simulink model "EST"  (R2023b)
settings: Solver=FixedStepAuto  StartTime=0.0  StopTime=stopt  FixedStep=deltat  MaxStep=0.05  RelTol=1e-3
InitFcn:
  | clear all;
  | close all;
  | clc;
  | 
  | % add the data and script directories
  | addpath('data','scripts');
  | 
  | % load the constants (units)
  | constants;
  | 
  | % load the simulation parameters
  | preprocessing;
StopFcn:
  | postprocessing;
values from neighbouring files (symbols this model uses):
  aElectricityDemandTransport = 0.01    [preprocessing.m]
  aExtraction = efficiency    [preprocessing.m]
  aHeatingDemandTransport = 0.01    [preprocessing.m]
  COP65 = 3    [preprocessing.m]
  COP80 = 2.48    [preprocessing.m]
  diameter = 1.2    [preprocessing.m]
  EStorageInitial = 10^5    (= 100000)    [preprocessing.m]
  EStorageMax = Tmax*HeatCapacity    (= 469413657.839)    [preprocessing.m]
  EStorageMin = Tmin*HeatCapacity    (= 352060243.38)    [preprocessing.m]
  HeatCapacity = WaterMass * SpecificHeat    (= 5867670.72299)    [preprocessing.m]
  HeatTransferCoefficient = 0.48    [preprocessing.m]
  InsulationThickness = 0.05    [preprocessing.m]
  SupplyVoltage = 230    [preprocessing.m]
  SupplyWireRestance = (WireLenght * ElectricalConductivity) / SupplyWireArea    (= 0.00530083402298)    [preprocessing.m]
  Tambient = 20    [preprocessing.m]
settings Model: Creator=joche  LastModifiedBy=20244239
settings DataIOCC: SaveFormat=Array  SaveOutput=off  ReturnWorkspaceOutputs=off
settings OptimizationCC: ReuseModelBlockBuffer=off
settings ModelReferenceCC: EnableRefExpFcnMdlSchedulingChecks=on

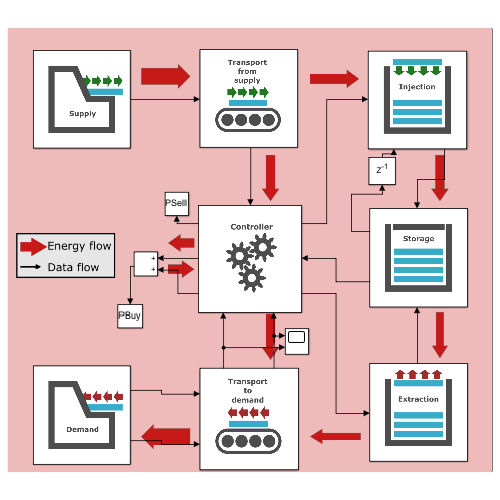
[thumbnail: Simulink's stored preview of the top-level diagram]
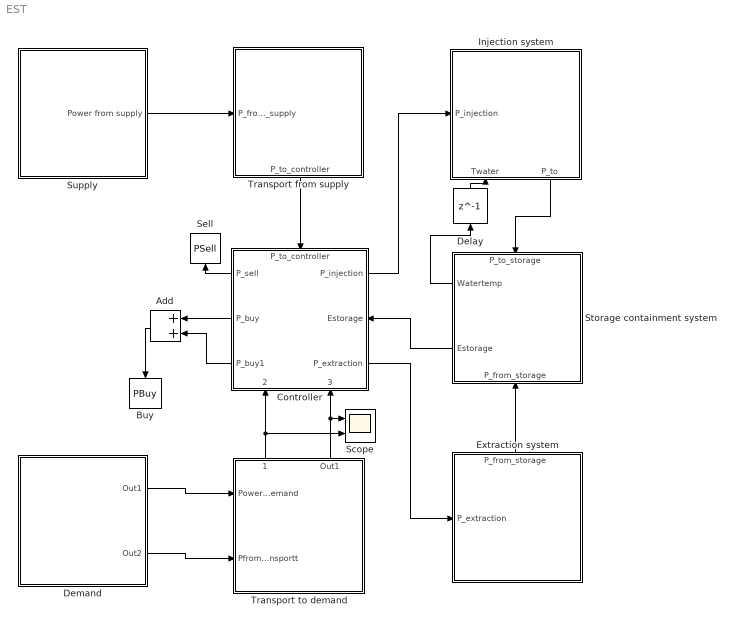
== system EST ==
  Add : Sum
  Buy : ToWorkspace  VariableName=PBuy  SampleTime=-1
  Controller : Subsystem
      settings: PortSchema="{\"entries\":[{\"content\":{\"sides\":[{\"content\":{\"connectorIds\":[\"Out3\",\"Out4\",\"Out5\"]},\"type\":\"ConnectorPlacement.EquallySpacedRectSide\",\"uuid\":\"4daf33ce-c96a-4783-b5c4-228eed953e01\"},{\"content\":{\"connectorIds\":[\"Out1\",\"In4\",\"Out2\"],\"side\":\"RIGHT\"},\"type\":\"ConnectorPlacement.EquallySpacedRectSide\",\"uuid\":\"e9942e50-8467-4af8-b79b-80636cbc76e5\"},{\"content\":{\"connectorIds\":[\"In1\"],\"side\":\"TOP\"},\"type\":\"ConnectorPlacement.EquallySpacedRectSide\",\"uuid\":\"f315e931-d69b-4751-b712-f89c6c81baeb\"},{\"content\":{\"connectorIds\":[\"In2\",\"In3\"],\"side\":\"BOTTOM\"},\"type\":\"ConnectorPlacement.EquallySpacedRectSide\",\"uuid\":\"44715ee6-5cd5-4669-bcb9-5ed7c869bdb3\"}]},\"type\":\"ConnectorPlacement.EquallySpacedConnector\",\"uuid\":\"fff48899-944b-4064-b7d7-ecc12144fb48\"}],\"packageUris\":[\"http://schema.mathworks.com/mf0/Connector/R2020b\"],\"version\":\"1.0\"}"
      mask Display: image('$imagefile'); % Use "Edit Image" on toolstrip to change.
  Delay : Delay  DelayLength=1  InitialCondition=0
  Demand : Subsystem
      mask Display: image('$imagefile'); % Use "Edit Image" on toolstrip to change.
  Extraction system : Subsystem
      settings: PortSchema="{\"entries\":[{\"content\":{\"sides\":[{\"content\":{\"connectorIds\":[]},\"type\":\"ConnectorPlacement.EquallySpacedRectSide\",\"uuid\":\"05c5933d-55fc-4e06-853f-fc26d42905f9\"},{\"content\":{\"connectorIds\":[\"In1\"],\"side\":\"RIGHT\"},\"type\":\"ConnectorPlacement.EquallySpacedRectSide\",\"uuid\":\"327426c5-31d5-498b-a2bd-83e49353408c\"},{\"content\":{\"connectorIds\":[],\"side\":\"TOP\"},\"type\":\"ConnectorPlacement.EquallySpacedRectSide\",\"uuid\":\"55306cf3-a3de-4385-a5ae-b8600ecdd5a2\"},{\"content\":{\"connectorIds\":[\"Out1\"],\"side\":\"BOTTOM\"},\"type\":\"ConnectorPlacement.EquallySpacedRectSide\",\"uuid\":\"08fcc9c3-40d3-4ac6-b914-dfeef6039ffb\"}]},\"type\":\"ConnectorPlacement.EquallySpacedConnector\",\"uuid\":\"cb35d5ba-e8c6-462c-b7b2-fe8356d4b0a1\"}],\"packageUris\":[\"http://schema.mathworks.com/mf0/Connector/R2020b\"],\"version\":\"1.0\"}"
      mask Display: image('$imagefile'); % Use "Edit Image" on toolstrip to change.
  Injection system : Subsystem
      settings: PortSchema="{\"entries\":[{\"content\":{\"sides\":[{\"content\":{},\"type\":\"ConnectorPlacement.EquallySpacedRectSide\",\"uuid\":\"05c5933d-55fc-4e06-853f-fc26d42905f9\"},{\"content\":{\"connectorIds\":[\"In2\"],\"side\":\"RIGHT\"},\"type\":\"ConnectorPlacement.EquallySpacedRectSide\",\"uuid\":\"327426c5-31d5-498b-a2bd-83e49353408c\"},{\"content\":{\"connectorIds\":[\"Out1\",\"In1\"],\"side\":\"TOP\"},\"type\":\"ConnectorPlacement.EquallySpacedRectSide\",\"uuid\":\"55306cf3-a3de-4385-a5ae-b8600ecdd5a2\"},{\"content\":{\"side\":\"BOTTOM\"},\"type\":\"ConnectorPlacement.EquallySpacedRectSide\",\"uuid\":\"08fcc9c3-40d3-4ac6-b914-dfeef6039ffb\"}]},\"type\":\"ConnectorPlacement.EquallySpacedConnector\",\"uuid\":\"cb35d5ba-e8c6-462c-b7b2-fe8356d4b0a1\"}],\"packageUris\":[\"http://schema.mathworks.com/mf0/Connector/R2020b\"],\"version\":\"1.0\"}"
      mask Display: image('$imagefile'); % Use "Edit Image" on toolstrip to change.
  Scope : Scope  NumInputPorts=2
  Sell : ToWorkspace  VariableName=PSell  SampleTime=-1
  Storage containment system : Subsystem
      settings: PortSchema="{\"entries\":[{\"content\":{\"sides\":[{\"content\":{\"connectorIds\":[\"Out1\",\"Out2\"]},\"type\":\"ConnectorPlacement.EquallySpacedRectSide\",\"uuid\":\"0ba48424-33b9-4934-970f-64fe5d8b070e\"},{\"content\":{\"side\":\"RIGHT\"},\"type\":\"ConnectorPlacement.EquallySpacedRectSide\",\"uuid\":\"9cde340f-8f39-4499-9a12-5e1623737660\"},{\"content\":{\"connectorIds\":[\"In1\"],\"side\":\"TOP\"},\"type\":\"ConnectorPlacement.EquallySpacedRectSide\",\"uuid\":\"2af8db04-7fd0-4902-8637-8dc00edb4598\"},{\"content\":{\"connectorIds\":[\"In2\"],\"side\":\"BOTTOM\"},\"type\":\"ConnectorPlacement.EquallySpacedRectSide\",\"uuid\":\"e21ea806-d777-41a3-a53f-556fae66854b\"}]},\"type\":\"ConnectorPlacement.EquallySpacedConnector\",\"uuid\":\"4e2ddb36-4db3-4ab4-858b-ebb8ccefeb1f\"}],\"packageUris\":[\"http://schema.mathworks.com/mf0/Connector/R2020b\"],\"version\":\"1.0\"}"
      mask Display: image('$imagefile'); % Use "Edit Image" on toolstrip to change.
  Supply : Subsystem
      mask Display: image('$imagefile'); % Use "Edit Image" on toolstrip to change.
  Transport from supply : Subsystem
      settings: PortSchema="{\"entries\":[{\"content\":{\"sides\":[{\"content\":{\"connectorIds\":[\"In1\"]},\"type\":\"ConnectorPlacement.EquallySpacedRectSide\",\"uuid\":\"31329006-3d36-4d93-9c44-7503a515d397\"},{\"content\":{\"connectorIds\":[],\"side\":\"RIGHT\"},\"type\":\"ConnectorPlacement.EquallySpacedRectSide\",\"uuid\":\"aba139c7-f9b6-4881-a56b-a4cbbedacd88\"},{\"content\":{\"connectorIds\":[],\"side\":\"TOP\"},\"type\":\"ConnectorPlacement.EquallySpacedRectSide\",\"uuid\":\"e683eb73-7a35-4160-9c39-da83856a6278\"},{\"content\":{\"connectorIds\":[\"Out1\"],\"side\":\"BOTTOM\"},\"type\":\"ConnectorPlacement.EquallySpacedRectSide\",\"uuid\":\"1170dd18-447c-437f-9043-6812c2877331\"}]},\"type\":\"ConnectorPlacement.EquallySpacedConnector\",\"uuid\":\"804af608-1d70-444f-af69-e05f19bf98f3\"}],\"packageUris\":[\"http://schema.mathworks.com/mf0/Connector/R2020b\"],\"version\":\"1.0\"}"
      mask Display: image('$imagefile'); % Use "Edit Image" on toolstrip to change.
  Transport to demand : Subsystem
      settings: PortSchema="{\"entries\":[{\"content\":{\"sides\":[{\"content\":{\"connectorIds\":[\"In1\",\"In2\"]},\"type\":\"ConnectorPlacement.EquallySpacedRectSide\",\"uuid\":\"03dcb471-e366-4ed9-a75b-6b53ae3db544\"},{\"content\":{\"side\":\"RIGHT\"},\"type\":\"ConnectorPlacement.EquallySpacedRectSide\",\"uuid\":\"6dd80e9d-b764-41ba-981e-efa62bb14601\"},{\"content\":{\"connectorIds\":[\"Out1\",\"Out2\"],\"side\":\"TOP\"},\"type\":\"ConnectorPlacement.EquallySpacedRectSide\",\"uuid\":\"5418711a-b225-492f-884c-10526dc9bc30\"}]},\"type\":\"ConnectorPlacement.EquallySpacedConnector\",\"uuid\":\"979ac05e-7956-4b8d-8463-5f461851369c\"}],\"packageUris\":[\"http://schema.mathworks.com/mf0/Connector/R2020b\"],\"version\":\"1.0\"}"
      mask Display: image('$imagefile'); % Use "Edit Image" on toolstrip to change.
  wires:
  Supply/1(Power from supply) -> Transport from supply/1(P_from_supply)
  Transport from supply/1(P_to_controller) -> Controller/1(P_to_controller)
  Transport to demand/1(P_from_controler) -> Scope/2, Controller/2(P_from_controller)
  Demand/1(Out1) -> Transport to demand/1(Power to demand)
  Controller/3(P_sell) -> Sell/1
  Controller/2(P_extraction) -> Extraction system/1(P_extraction)
  Injection system/1(P_to) -> Storage containment system/1(P_to_storage)
  Extraction system/1(P_from_storage) -> Storage containment system/2(P_from_storage)
  Controller/1(P_injection) -> Injection system/2(P_injection)
  Controller/4(P_buy) -> Add/1
  Demand/2(Out2) -> Transport to demand/2(PfromElectricityDemandTransportt)
  Transport to demand/2(Out1) -> Controller/3(PElectricityFromController), Scope/1
  Controller/5(P_buy1) -> Add/2
  Add/1 -> Buy/1
  Storage containment system/2(Estorage) -> Controller/4(Estorage)
  Storage containment system/1(Watertemp) -> Delay/1
  Delay/1 -> Injection system/1(Twater)

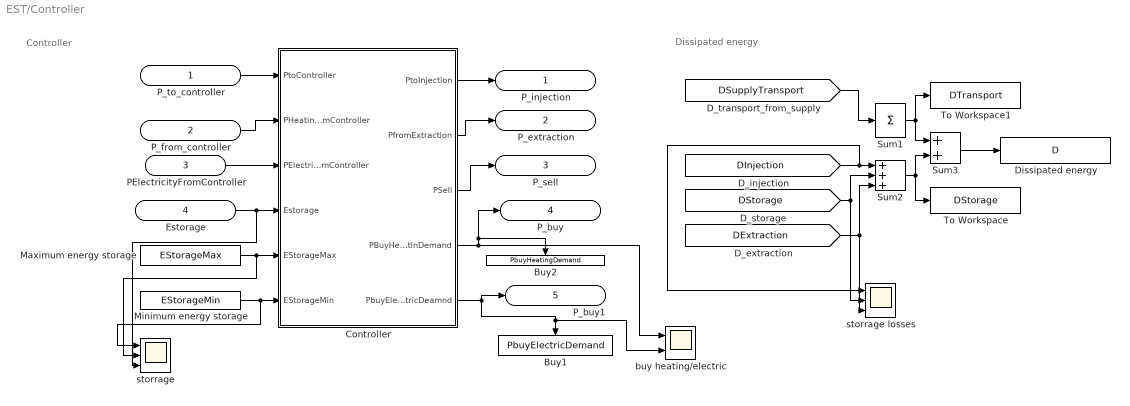
== system EST/Controller ==
  note: Dissipated energy
  note: Controller
  P_to_controller : Inport
  P_from_controller : Inport  Port=2
  PElectricityFromController : Inport  Port=3
  Estorage : Inport  Port=4
  Buy1 : ToWorkspace  VariableName=PbuyElectricDemand  SampleTime=-1
  Buy2 : ToWorkspace  VariableName=PbuyHeatingDemand  SampleTime=-1
  Controller : MATLAB Function  TreatAsAtomicUnit=on
  Dissipated energy : ToWorkspace  VariableName=D  SampleTime=-1
  Maximum energy storage : Constant  Value=EStorageMax
  Minimum energy storage : Constant  Value=EStorageMin
  Sum1 : Sum  Inputs=+
  Sum2 : Sum  Inputs=+++
  Sum3 : Sum
  To Workspace : ToWorkspace  VariableName=DStorage  SampleTime=-1
  To Workspace1 : ToWorkspace  VariableName=DTransport  SampleTime=-1
  buy heating/electric : Scope  NumInputPorts=2
  storrage : Scope  NumInputPorts=3
  storrage losses : Scope  NumInputPorts=3
  P_injection : Outport
  P_extraction : Outport  Port=2
  P_sell : Outport  Port=3
  P_buy : Outport  Port=4
  P_buy1 : Outport  Port=5
  wires:
  P_from_controller/1 -> Controller/2(PHeatingfromController)
  Controller/2(PfromExtraction) -> P_extraction/1
  Controller/3(PSell) -> P_sell/1
  Controller/4(PBuyHeatinDemand) -> buy heating/electric/1, P_buy/1, Buy2/1
  Minimum energy storage/1 -> storrage/1, Controller/6(EStorageMin)
  Maximum energy storage/1 -> storrage/2, Controller/5(EStorageMax)
  P_to_controller/1 -> Controller/1(PtoController)
  Controller/1(PtoInjection) -> P_injection/1
  Estorage/1 -> storrage/3, Controller/4(Estorage)
  [DSupplyTransport] -> Sum1/1
  [DInjection] -> storrage losses/1, Sum2/1
  [DStorage] -> Sum2/2, storrage losses/2
  [DExtraction] -> Sum2/3, storrage losses/3
  Sum2/1 -> To Workspace/1, Sum3/2
  Sum1/1 -> To Workspace1/1, Sum3/1
  Sum3/1 -> Dissipated energy/1
  PElectricityFromController/1 -> Controller/3(PElectricityFromController)
  Controller/5(PbuyElectricDeamnd) -> buy heating/electric/2, Buy1/1, P_buy1/1

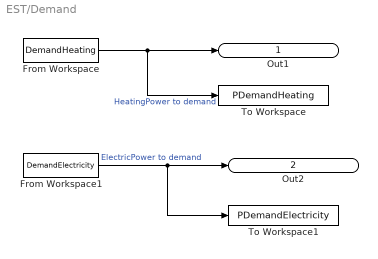
== system EST/Demand ==
  From Workspace : FromWorkspace  VariableName=DemandHeating  OutputAfterFinalValue=Setting to zero
  From Workspace1 : FromWorkspace  VariableName=DemandElectricity  OutputAfterFinalValue=Setting to zero
  To Workspace : ToWorkspace  VariableName=PDemandHeating  SampleTime=-1
  To Workspace1 : ToWorkspace  VariableName=PDemandElectricity  SampleTime=-1
  Out1 : Outport
  Out2 : Outport  Port=2
  wires:
  From Workspace/1 -> To Workspace/1, Out1/1  "HeatingPower to demand"
  From Workspace1/1 -> To Workspace1/1, Out2/1  "ElectricPower to demand"

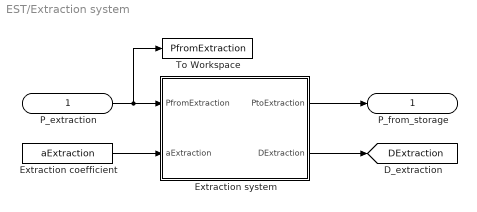
== system EST/Extraction system ==
  P_extraction : Inport
  Extraction coefficient : Constant  Value=aExtraction
  Extraction system : MATLAB Function  TreatAsAtomicUnit=on
  To Workspace : ToWorkspace  VariableName=PfromExtraction  SampleTime=-1
  P_from_storage : Outport
  tag scope: DExtraction=global
  wires:
  P_extraction/1 -> To Workspace/1, Extraction system/1(PfromExtraction)
  Extraction system/1(PtoExtraction) -> P_from_storage/1
  Extraction coefficient/1 -> Extraction system/2(aExtraction)
  Extraction system/2(DExtraction) -> [DExtraction]

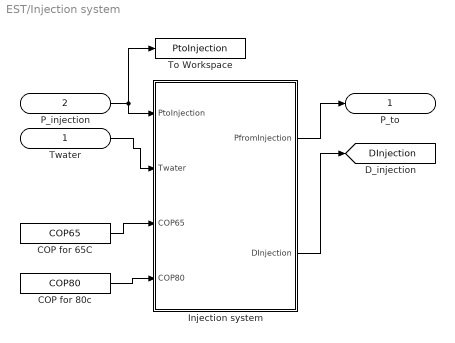
== system EST/Injection system ==
  Twater : Inport
  P_injection : Inport  Port=2
  COP for 65C : Constant  Value=COP65
  COP for 80c : Constant  Value=COP80
  Injection system : MATLAB Function  TreatAsAtomicUnit=on
  To Workspace : ToWorkspace  VariableName=PtoInjection  SampleTime=-1
  P_to : Outport
  tag scope: DInjection=global
  wires:
  P_injection/1 -> To Workspace/1, Injection system/1(PtoInjection)
  Injection system/1(PfromInjection) -> P_to/1
  Injection system/2(DInjection) -> [DInjection]
  COP for 65C/1 -> Injection system/3(COP65)
  COP for 80c/1 -> Injection system/4(COP80)
  Twater/1 -> Injection system/2(Twater)

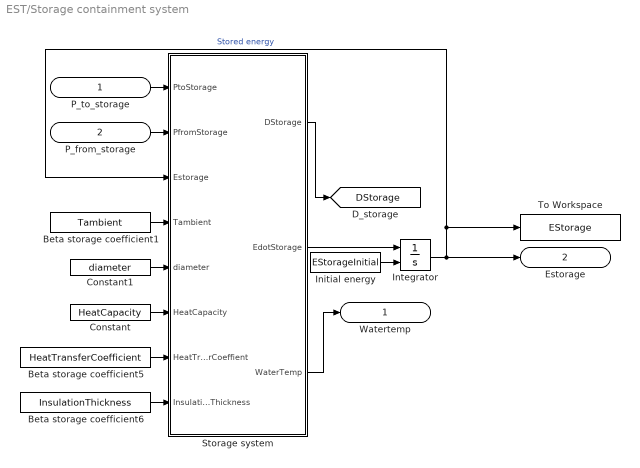
== system EST/Storage containment system ==
  P_to_storage : Inport
  P_from_storage : Inport  Port=2
  Beta storage coefficient1 : Constant  Value=Tambient
  Beta storage coefficient5 : Constant  Value=HeatTransferCoefficient
  Beta storage coefficient6 : Constant  Value=InsulationThickness
  Constant : Constant  Value=HeatCapacity
  Constant1 : Constant  Value=diameter
  Initial energy : Constant  Value=EStorageInitial
  Integrator : Integrator  InitialConditionSource=external
  Storage system : MATLAB Function  TreatAsAtomicUnit=on
  To Workspace : ToWorkspace  VariableName=EStorage  SampleTime=-1
  Watertemp : Outport
  Estorage : Outport  Port=2
  tag scope: DStorage=global
  wires:
  P_from_storage/1 -> Storage system/2(PfromStorage)
  P_to_storage/1 -> Storage system/1(PtoStorage)
  Initial energy/1 -> Integrator/2
  Integrator/1 -> Storage system/3(Estorage), To Workspace/1, Estorage/1  "Stored energy"
  Storage system/1(DStorage) -> [DStorage]
  Storage system/2(EdotStorage) -> Integrator/1
  Beta storage coefficient1/1 -> Storage system/4(Tambient)
  Beta storage coefficient5/1 -> Storage system/7(HeatTransferCoeffient)
  Beta storage coefficient6/1 -> Storage system/8(InsulationThickness)
  Constant/1 -> Storage system/6(HeatCapacity)
  Storage system/3(WaterTemp) -> Watertemp/1
  Constant1/1 -> Storage system/5(diameter)

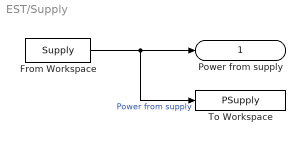
== system EST/Supply ==
  From Workspace : FromWorkspace  VariableName=Supply  OutputAfterFinalValue=Setting to zero
  To Workspace : ToWorkspace  VariableName=PSupply  SampleTime=-1
  Power from supply : Outport
  wires:
  From Workspace/1 -> To Workspace/1, Power from supply/1  "Power from supply"

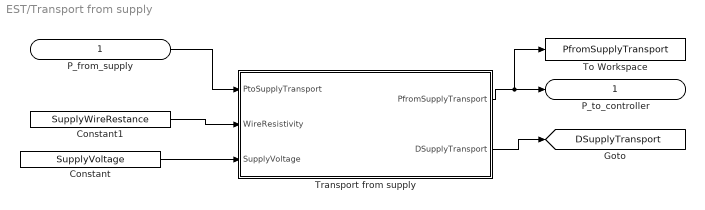
== system EST/Transport from supply ==
  P_from_supply : Inport
  Constant : Constant  Value=SupplyVoltage  VectorParams1D=off  SampleTime=-1
  Constant1 : Constant  Value=SupplyWireRestance  SampleTime=-1
  To Workspace : ToWorkspace  VariableName=PfromSupplyTransport  SampleTime=-1
  Transport from supply : MATLAB Function  TreatAsAtomicUnit=on
  P_to_controller : Outport
  tag scope: DSupplyTransport=global
  wires:
  Constant/1 -> Transport from supply/3(SupplyVoltage)
  P_from_supply/1 -> Transport from supply/1(PtoSupplyTransport)
  Transport from supply/1(PfromSupplyTransport) -> To Workspace/1, P_to_controller/1
  Transport from supply/2(DSupplyTransport) -> [DSupplyTransport]
  Constant1/1 -> Transport from supply/2(WireResistivity)

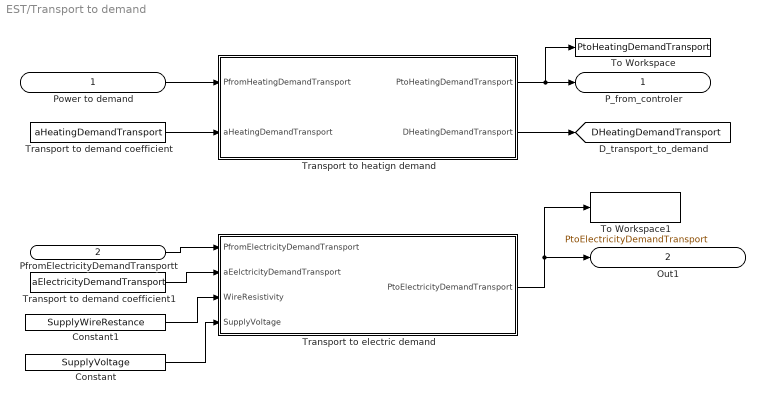
== system EST/Transport to demand ==
  Power to demand : Inport
  PfromElectricityDemandTransportt : Inport  Port=2
  Constant : Constant  Value=SupplyVoltage  VectorParams1D=off  SampleTime=-1
  Constant1 : Constant  Value=SupplyWireRestance  SampleTime=-1
  To Workspace : ToWorkspace  VariableName=PtoHeatingDemandTransport  SampleTime=-1
  To Workspace1 : ToWorkspace  VariableName=PtoElectricityDemandTransport  SampleTime=-1
  Transport to demand coefficient : Constant  Value=aHeatingDemandTransport
  Transport to demand coefficient1 : Constant  Value=aElectricityDemandTransport
  Transport to electric demand : MATLAB Function  TreatAsAtomicUnit=on
  Transport to heatign demand : MATLAB Function  TreatAsAtomicUnit=on
  P_from_controler : Outport
  Out1 : Outport  Port=2
  tag scope: DHeatingDemandTransport=global
  wires:
  Transport to demand coefficient/1 -> Transport to heatign demand/2(aHeatingDemandTransport)
  Power to demand/1 -> Transport to heatign demand/1(PfromHeatingDemandTransport)
  Transport to heatign demand/1(PtoHeatingDemandTransport) -> To Workspace/1, P_from_controler/1
  Transport to heatign demand/2(DHeatingDemandTransport) -> [DHeatingDemandTransport]
  Transport to demand coefficient1/1 -> Transport to electric demand/2(aEelctricityDemandTransport)
  PfromElectricityDemandTransportt/1 -> Transport to electric demand/1(PfromElectricityDemandTransport)
  Transport to electric demand/1(PtoElectricityDemandTransport) -> To Workspace1/1, Out1/1
  Constant1/1 -> Transport to electric demand/3(WireResistivity)
  Constant/1 -> Transport to electric demand/4(SupplyVoltage)

== matlab function EST/Transport to demand/Transport to heatign demand ==
  data: PfromHeatingDemandTransport input; PtoHeatingDemandTransport output; DHeatingDemandTransport output; aHeatingDemandTransport input
function [PtoHeatingDemandTransport, DHeatingDemandTransport] = demandTransport(PfromHeatingDemandTransport,aHeatingDemandTransport)

    DHeatingDemandTransport = aHeatingDemandTransport / (1-aHeatingDemandTransport) * PfromHeatingDemandTransport;
    PtoHeatingDemandTransport = PfromHeatingDemandTransport + DHeatingDemandTransport;

== matlab function EST/Injection system/Injection system ==
  data: PtoInjection input; Twater input; PfromInjection output; DInjection output; COP65 input; COP80 input
function [PfromInjection, DInjection] = injection(PtoInjection, Twater, COP65, COP80)
    if Twater<65
        COP = COP65;
    else 
        COP = (COP80-COP65)/15*(Twater-65)+COP65;
    end
    DInjection = 0;
    PfromInjection = PtoInjection*COP;

== matlab function EST/Transport from supply/Transport from supply ==
  data: PtoSupplyTransport input; PfromSupplyTransport output; WireResistivity input; DSupplyTransport output; SupplyVoltage input
function [PfromSupplyTransport, DSupplyTransport]= supplyTransport(PtoSupplyTransport, WireResistivity ,SupplyVoltage)
    Current = PtoSupplyTransport/SupplyVoltage;
    Ploss = WireResistivity * Current^2;

    DSupplyTransport = Ploss;
    PfromSupplyTransport = PtoSupplyTransport - DSupplyTransport;

== matlab function EST/Controller/Controller ==
  data: PtoInjection output; PfromExtraction output; PSell output; PBuyHeatinDemand output; PtoController input; PHeatingfromController input; PElectricityFromController input; Estorage input; EStorageMax input; EStorageMin input; PbuyElectricDeamnd output
function [PtoInjection, PfromExtraction, PSell, PBuyHeatinDemand,PbuyElectricDeamnd] = controller(PtoController, PHeatingfromController, PElectricityFromController, Estorage, EStorageMax, EStorageMin)
    
    %% Reset all outputs to zero
    PBuyHeatinDemand = 0;
    PtoInjection = 0;
    PSell = 0;
    PbuyElectricDeamnd = 0;

    %% Handle electric power from solar vs need
    if PElectricityFromController < PtoController
        if Estorage < EStorageMax
            PtoInjection = PtoController - PElectricityFromController;
        else
            PSell = PtoController - PElectricityFromController;
        end 
    else
        PbuyElectricDeamnd = PElectricityFromController - PtoController;
    end

    %% Handle heating demand from storage or external bought energy
    if Estorage > EStorageMin
        PfromExtraction = PHeatingfromController;
    else %%Not enough energy in storage to covver demand
        PBuyHeatinDemand = PHeatingfromController;
        PtoInjection = PtoInjection + PHeatingfromController;
        PfromExtraction = PHeatingfromController;
    end
end



%% Currently unused code, kept in case it is referred to in future
    %{
    if PsurplusSolar <= 0 %buying electricity if electric consumption isn't covered 
        PBuy = PsurplusSolar;
    else % Power surplus (so more supply than electric usage)
        PBuy = 0;
        %% storre all extra energy 

        % Check if storage system is not full
        if EStorage < EStrorageMax 

            PtoInjection = PsurplusSolar;

        % if storrage system is full sell the surplus
        else
            PtoInjection = 0;
            PSell = PsurplusSolar;
        end    
        
    end 

    %all heating goes through the heatpump and the heat storrage 
    PfromExtraction = PHeatingfromController;

    if EStorage < 0
        PBuy = PBuy-EStorage;
        PtoInjection = PtoInjection + PBuy;
    end
    %}

== matlab function EST/Extraction system/Extraction system ==
  data: PfromExtraction input; PtoExtraction output; aExtraction input; DExtraction output
function [PtoExtraction, DExtraction] = extraction(PfromExtraction, aExtraction)
    DExtraction = aExtraction / (1-aExtraction) * PfromExtraction;
    PtoExtraction = PfromExtraction + DExtraction;

== matlab function EST/Storage containment system/Storage system ==
  data: DStorage output; EdotStorage output; PtoStorage input; PfromStorage input; Estorage input; Tambient input; diameter input; HeatCapacity input; HeatTransferCoeffient input; InsulationThickness input; WaterTemp output
function [DStorage, EdotStorage, WaterTemp]= ...
    Storage(PtoStorage, PfromStorage, Estorage, Tambient, diameter, HeatCapacity, HeatTransferCoeffient, InsulationThickness)

    WaterTemp = Estorage/(HeatCapacity);
    Area = pi * diameter;

    DStorage = (WaterTemp-Tambient)*Area*HeatTransferCoeffient/InsulationThickness;
    EdotStorage = PtoStorage - PfromStorage - DStorage;

== matlab function EST/Transport to demand/Transport to electric demand ==
  data: PfromElectricityDemandTransport input; PtoElectricityDemandTransport output; aEelctricityDemandTransport input; WireResistivity input; SupplyVoltage input
function PtoElectricityDemandTransport  = demandTransport(PfromElectricityDemandTransport,aEelctricityDemandTransport,WireResistivity,SupplyVoltage)

    Current = PfromElectricityDemandTransport/SupplyVoltage;
    lossWire = WireResistivity * Current^2;

    PfromElectricityDemandTransport = PfromElectricityDemandTransport * (1 - lossWire);

    DElectricityDemandTransport = aEelctricityDemandTransport / (1-aEelctricityDemandTransport) * PfromElectricityDemandTransport;
    PtoElectricityDemandTransport = PfromElectricityDemandTransport - DElectricityDemandTransport;
